simulink model "OpenLoopBruceMotor"  (R2024b)
settings: Solver=VariableStepAuto  StartTime=0.0  StopTime=5  RelTol=1e-3
InitFcn:
  | MotorSimulationParams
values from neighbouring files (symbols this model uses):
  B_PMSM = 0    [MotorSimulationParams.m]
  F_PMSM = 1e-3    (= 0.001)    [MotorSimulationParams.m]
  J_PMSM = 1.879e-6    (= 1.879e-06)    [MotorSimulationParams.m]
  Load_Torque = 0    [MotorSimulationParams.m]
  Pole_Pairs = 1    [MotorSimulationParams.m]
  Rline = 1e-3    (= 0.001)    [MotorSimulationParams.m]
  Rs = 312e-3    (= 0.312)    [MotorSimulationParams.m]
  Tramp = 1    [MotorSimulationParams.m]
  Vsource = 10    [MotorSimulationParams.m]
  Wrated = Rated_Speed/60*2*pi    (= 282.743338823)    [MotorSimulationParams.m]
undefined symbols (not defined in the file or in its folder): Lline
libraries: spsGroundLib x6, spsVoltageMeasurementLib x6, spsHalfBridgeConverterLib x3, spsPWMGenerator2LevelLib x3, spsThreePhaseSeriesRLCBranchLib x2, spsCurrentMeasurementLib x1, spsDCVoltageSourceLib x1, spsPermanentMagnetSynchronousMachineLib x1, spsThreePhaseProgrammableVoltageSourceLib x1, spsdq0toabcLib x1, sps_lib x1
settings Model: Creator=pickl  LastModifiedBy=pickl
settings SolverCC: ZeroCrossAlgorithm=Adaptive
settings DebuggingCC: MaskedZcDiagnostic=none  IgnoredZcDiagnostic=none

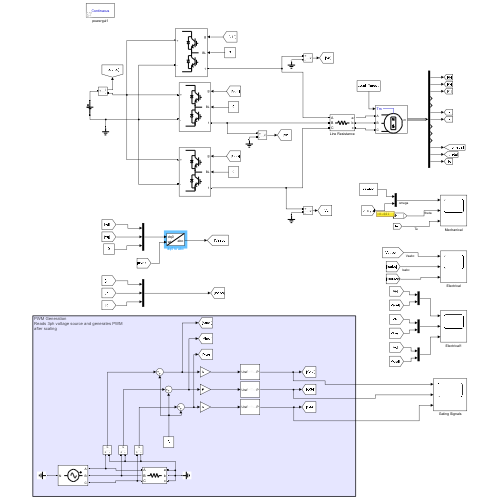
[thumbnail: Simulink's stored preview of the top-level diagram]
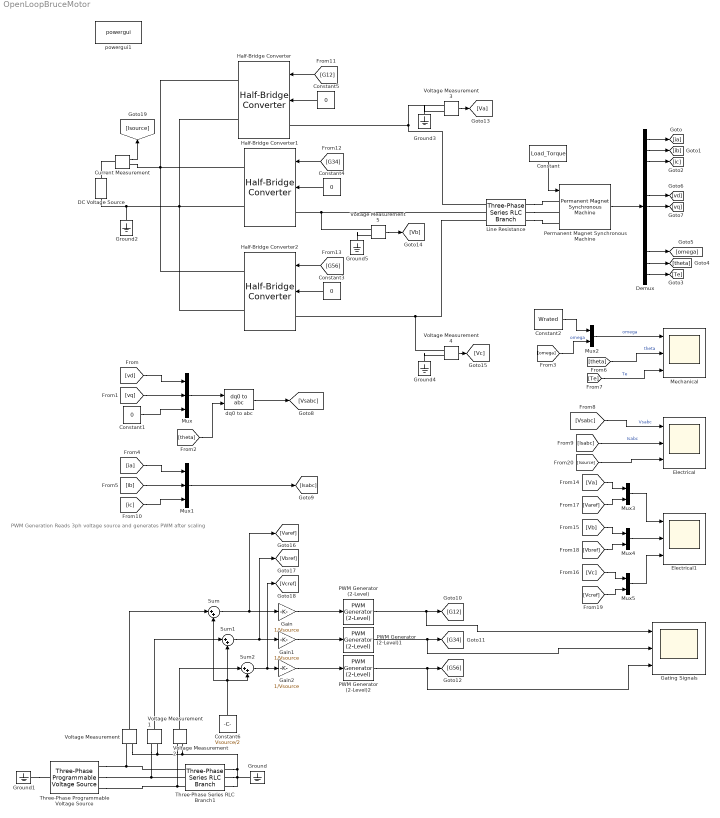
== system OpenLoopBruceMotor ==
  note: PWM Generation
      | Reads 3ph voltage source and generates PWM
      | after scaling
  Constant : Constant  Value=Load_Torque
  Constant{1,3..5} (4 alike) : Constant  Value=0
  Constant2 : Constant  Value=Wrated
  Constant6 : Constant  Value=Vsource/2
  Current Measurement : spsCurrentMeasurementLib/Current Measurement  PhasorSimulation=off  OutputType=Complex  PSBequivalent=0
  DC Voltage Source : spsDCVoltageSourceLib/DC Voltage Source  Amplitude=Vsource  Measurements=None
  Demux : Demux  Outputs=13
  Electrical : Scope  NumInputPorts=3
  Electrical1 : Scope  NumInputPorts=3
  Gain : Gain  Gain=1/Vsource
  Gain1 : Gain  Gain=1/Vsource
  Gain2 : Gain  Gain=1/Vsource
  Gating Signals : Scope  NumInputPorts=3
  Ground{,1..5} (6 alike) : spsGroundLib/Ground  LConnTagsString=a
  Half-Bridge Converter : spsHalfBridgeConverterLib/Half-Bridge Converter  ModelType=Switching function  Ron=1e-3  Rs=1e6  Cs=inf  Vforward=[0,0]  Ron_Diode=Ron  Rs_Diode=1e6  Cs_Diode=inf  Vf_Diode=Vds  Rs_CurrentSource=inf  Ron_ACsource=10e-3
      settings: LibrarySourceBlock=sps_lib/Power Electronics/Half-Bridge Converter
  Half-Bridge Converter1 : spsHalfBridgeConverterLib/Half-Bridge Converter  ModelType=Switching function  Ron=1e-3  Rs=1e6  Cs=inf  Vforward=[0,0]  Ron_Diode=Ron  Rs_Diode=1e6  Cs_Diode=inf  Vf_Diode=Vds  Rs_CurrentSource=inf  Ron_ACsource=10e-3
      settings: LibrarySourceBlock=sps_lib/Power Electronics/Half-Bridge Converter
  Half-Bridge Converter2 : spsHalfBridgeConverterLib/Half-Bridge Converter  ModelType=Switching function  Ron=1e-3  Rs=1e6  Cs=inf  Vforward=[0,0]  Ron_Diode=Ron  Rs_Diode=1e6  Cs_Diode=inf  Vf_Diode=Vds  Rs_CurrentSource=inf  Ron_ACsource=10e-3
      settings: LibrarySourceBlock=sps_lib/Power Electronics/Half-Bridge Converter
  Line Resistance : spsThreePhaseSeriesRLCBranchLib/Three-Phase Series RLC Branch  LConnTagsString=A|B|C  RConnTagsString=A|B|C  BranchType=R  Resistance=Rline  Inductance=Lline  Capacitance=1e-6  Measurements=None
  Mechanical : Scope  NumInputPorts=3
  Mux : Mux  Inputs=3
  Mux1 : Mux  Inputs=3
  Mux{2..5} (4 alike) : Mux  Inputs=2
  PWM Generator (2-Level) : spsPWMGenerator2LevelLib/PWM Generator (2-Level)  ModulatorType=Single-phase half-bridge (2 pulses)  ModulatorMode=Unsynchronized  Fc=fsw  Pc=0  nF=27  MinMax=[0, 1]  SamplingTechnique=Symmetrical regular (single edge)  ModulatingSignals=off  m=0.8  Freq=60  Phase=0  Ts=0  ShowCarrierOutport=off
  PWM Generator (2-Level)1 : spsPWMGenerator2LevelLib/PWM Generator (2-Level)  ModulatorType=Single-phase half-bridge (2 pulses)  ModulatorMode=Unsynchronized  Fc=fsw  Pc=0  nF=27  MinMax=[0, 1]  SamplingTechnique=Symmetrical regular (single edge)  ModulatingSignals=off  m=0.8  Freq=60  Phase=0  Ts=0  ShowCarrierOutport=off
  PWM Generator (2-Level)2 : spsPWMGenerator2LevelLib/PWM Generator (2-Level)  ModulatorType=Single-phase half-bridge (2 pulses)  ModulatorMode=Unsynchronized  Fc=fsw  Pc=0  nF=27  MinMax=[0, 1]  SamplingTechnique=Symmetrical regular (single edge)  ModulatingSignals=off  m=0.8  Freq=60  Phase=0  Ts=0  ShowCarrierOutport=off
  Permanent Magnet Synchronous Machine : spsPermanentMagnetSynchronousMachineLib/Permanent Magnet Synchronous Machine  NbPhases=3  FluxDistribution=Sinusoidal  RotorType=Round  MechanicalLoad=Torque Tm  PresetModel=No  ShowDetailedParameters=on  MeasurementBus=off  Resistance=Rs  Inductance=8.5e-3  dqInductances=[8.5e-3,8.5e-3]  La=Lq  MachineConstant=Flux linkage established by magnets (V.s)  Flux=lambda  VoltageCst=0.087987  TorqueCst=0.00072765  Flat=120  Mechanical=[J_PMSM, F_PMSM, Pole_Pairs, B_PMSM]  PolePairs=2  InitialConditions=[0,0, 0,0]  InitialConditions5ph=[0 0 0 0 0 0]  RefAngle=90 degrees behind phase A axis (modified Park)  IterativeDiscreteModel=Trapezoidal non iterative  TsBlock=-1  TsPowergui=0
  Sum : Sum  Inputs=|++
  Sum1 : Sum  Inputs=|++
  Sum2 : Sum  Inputs=|++
  Three-Phase Programmable Voltage Source : spsThreePhaseProgrammableVoltageSourceLib/Three-Phase Programmable Voltage Source  PositiveSequence=[Vsource/2*(sqrt(3/2)) 0 0]  VariationEntity=Frequency  VariationType=Table of time-amplitude pairs  VariationTypeAlt=Ramp  VariationStep=0.5  VariationRate=Frated/Tramp  VariationMagnitude=0.3  VariationFrequency=2  VariationTiming=[0.2 Tramp+0.2]  VariationPhaseA=off  Amplitudes=[1 0.8 1.2 1.0]  TimeValues=[0 0.1 0.15 0.2]  HarmonicGeneration=off  HarmonicA=[3 0.2 -25 0]  HarmonicB=[2 0.15 35 2]  Timing="[0.05  3]"  BusType=swing  Pref=0  Qref=0  Qmin=-inf  Qmax=inf
  Three-Phase Series RLC Branch1 : spsThreePhaseSeriesRLCBranchLib/Three-Phase Series RLC Branch  LConnTagsString=A|B|C  RConnTagsString=A|B|C  BranchType=R  Resistance=Rline  Inductance=1e-3  Capacitance=1e-6  Measurements=None
  Voltage Measurement{,1..5} (6 alike) : spsVoltageMeasurementLib/Voltage Measurement  PhasorSimulation=off  OutputType=Complex  PSBequivalent=0
  dq0 to abc : spsdq0toabcLib/dq0 to abc  Alignment=Aligned with phase A axis
  powergui1 : sps_lib/powergui  Priority=1  SimulationMode=Continuous  SampleTime=50e-6  frequency=60  Iterations=50  frequencyindice=0  Pbase=100e6  ErrMax=1e-4  UnitsV=kV  UnitsW=MW  buscounter=0  FunctionMessages=off  echomessages=off  EnableUseOfTLC=off  CurrentSourceSwitches=off  DisableSnubberDevices=off  DisableRonSwitches=off  DisableVfSwitches=off  DisplayEquations=off  AutomaticDiscreteSolvers=off  SolverType=Tustin/Backward Euler (TBE)  Interpol=off  ExternalGateDelay=off  methode=off  Ts=100  x0status=blocks  SPID=on  SwTol=0  HookPort=off  NonlinearTolerance=1e-4  nMaxIteration=100  ContinueOnMaxIteration=off  RestoreLinks=warning  ResistiveCurrentMeasurement=off  Frange=[0:2:500]  Ylog=off  Xlog=on  ShowGrid=off  save=off  variable=ZData  structure=0  ZoomFFT=off  StartTime=0.0  cycles=1  DisplayStyle=1  fundamental=60  FreqAxis=off  MaxFrequency=1000  frequencyindicesteady=1  RmsSteady=1  display=off
  wires:
  Constant/1 -> Permanent Magnet Synchronous Machine/1
  Permanent Magnet Synchronous Machine/1 -> Demux/1
  Demux/1 -> [ia]
  Demux/2 -> [ib]
  Demux/3 -> [ic]
  Demux/13 -> [Te]
  Demux/12 -> [theta]
  Demux/11 -> [omega]
  Demux/6 -> [vd]
  Demux/7 -> [vq]
  [vq] -> Mux/2
  Constant1/1 -> Mux/3
  [vd] -> Mux/1
  Mux/1 -> dq0 to abc/1
  [theta] -> dq0 to abc/2
  dq0 to abc/1 -> [Vsabc]
  [ib] -> Mux1/2
  [ic] -> Mux1/3
  [ia] -> Mux1/1
  Mux1/1 -> [Isabc]
  [theta] -> Mechanical/2  "theta"
  [Te] -> Mechanical/3  "Te"
  [Vsabc] -> Electrical/1  "Vsabc"
  [Isabc] -> Electrical/2  "Isabc"
  Mux2/1 -> Mechanical/1  "omega"
  Constant2/1 -> Mux2/1
  [omega] -> Mux2/2  "omega"
  [G34] -> Half-Bridge Converter1/1
  Constant3/1 -> Half-Bridge Converter2/2
  [G56] -> Half-Bridge Converter2/1
  [G12] -> Half-Bridge Converter/1
  Constant4/1 -> Half-Bridge Converter1/2
  Constant5/1 -> Half-Bridge Converter/2
  Voltage Measurement3/1 -> [Va]
  Voltage Measurement5/1 -> [Vb]
  Voltage Measurement4/1 -> [Vc]
  [Va] -> Mux3/1
  [Varef] -> Mux3/2
  [Vb] -> Mux4/1
  [Vbref] -> Mux4/2
  [Vc] -> Mux5/1
  [Vcref] -> Mux5/2
  Mux4/1 -> Electrical1/2
  Mux3/1 -> Electrical1/1
  Mux5/1 -> Electrical1/3
  Constant6/1 -> Sum1/2, Sum2/2, Sum/2
  Voltage Measurement/1 -> Sum/1
  Voltage Measurement1/1 -> Sum1/1
  Voltage Measurement2/1 -> Sum2/1
  Sum/1 -> [Varef], Gain/1
  Sum1/1 -> [Vbref], Gain1/1
  Sum2/1 -> [Vcref], Gain2/1
  Gain/1 -> PWM Generator (2-Level)/1
  Gain1/1 -> PWM Generator (2-Level)1/1
  Gain2/1 -> PWM Generator (2-Level)2/1
  PWM Generator (2-Level)/1 -> Gating Signals/1, [G12]
  PWM Generator (2-Level)1/1 -> Gating Signals/2, [G34]
  PWM Generator (2-Level)2/1 -> Gating Signals/3, [G56]
  Current Measurement/1 -> [Isource]
  [Isource] -> Electrical/3
  connections:
  Line Resistance/RConn2 -- Permanent Magnet Synchronous Machine/LConn2
  Line Resistance/RConn1 -- Permanent Magnet Synchronous Machine/LConn1
  Line Resistance/RConn3 -- Permanent Magnet Synchronous Machine/LConn3
  Line Resistance/LConn2 -- Half-Bridge Converter1/LConn1 -- Voltage Measurement5/LConn1
  Line Resistance/LConn1 -- Voltage Measurement3/LConn1 -- Half-Bridge Converter/LConn1
  Line Resistance/LConn3 -- Voltage Measurement4/LConn1 -- Half-Bridge Converter2/LConn1
  Half-Bridge Converter1/RConn1 -- Half-Bridge Converter/RConn1 -- Current Measurement/RConn1 -- Half-Bridge Converter2/RConn1
  DC Voltage Source/LConn1 -- Ground2/LConn1 -- Half-Bridge Converter2/RConn2 -- Half-Bridge Converter/RConn2 -- Half-Bridge Converter1/RConn2
  Ground3/LConn1 -- Voltage Measurement3/LConn2
  Ground4/LConn1 -- Voltage Measurement4/LConn2
  Ground5/LConn1 -- Voltage Measurement5/LConn2
  Three-Phase Series RLC Branch1/RConn1 -- Voltage Measurement2/LConn2 -- Voltage Measurement1/LConn2 -- Voltage Measurement/LConn2 -- Three-Phase Series RLC Branch1/RConn3 -- Three-Phase Series RLC Branch1/RConn2 -- Ground/LConn1
  Three-Phase Programmable Voltage Source/RConn3 -- Voltage Measurement2/LConn1 -- Three-Phase Series RLC Branch1/LConn3
  Ground1/LConn1 -- Three-Phase Programmable Voltage Source/LConn1
  Three-Phase Programmable Voltage Source/RConn1 -- Voltage Measurement/LConn1 -- Three-Phase Series RLC Branch1/LConn1
  Three-Phase Programmable Voltage Source/RConn2 -- Voltage Measurement1/LConn1 -- Three-Phase Series RLC Branch1/LConn2
  Current Measurement/LConn1 -- DC Voltage Source/RConn1
